simulink model "pinv_64x32"  (R2024a)
settings: Solver=VariableStepAuto  StartTime=0.0  StopTime=16384  RelTol=1e-3
PostLoadFcn:
  | xmcCheckSlxPath(bdroot)
  | setup
values from neighbouring files (symbols this model uses):
  MATMULT_RH_INPUT1_SAMPLES = MATMULT_INPUT_SAMPLES    (= 2048)    [setup.m]
undefined symbols (not defined in the file or in its folder): S, vsva2197, xcvc1902
libraries: aieBasic x7, dspsrcs4 x1, vmcUtilities x1, dspinverses x1, aieUtilities x1
settings Model: Creator=viswanad  LastModifiedBy=sdegala
settings SolverCC: AlgebraicLoopSolver=TrustRegion
settings DebuggingCC: UnconnectedInputMsg=warning  UnconnectedOutputMsg=warning  UnconnectedLineMsg=warning
settings ModelReferenceCC: EnableRefExpFcnMdlSchedulingChecks=on
settings RTWCC: GPUComputeCapability=3.5  DLArmComputeVersion=19.05

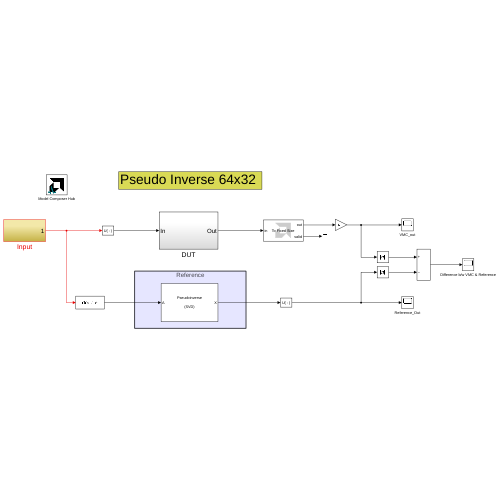
[thumbnail: Simulink's stored preview of the top-level diagram]
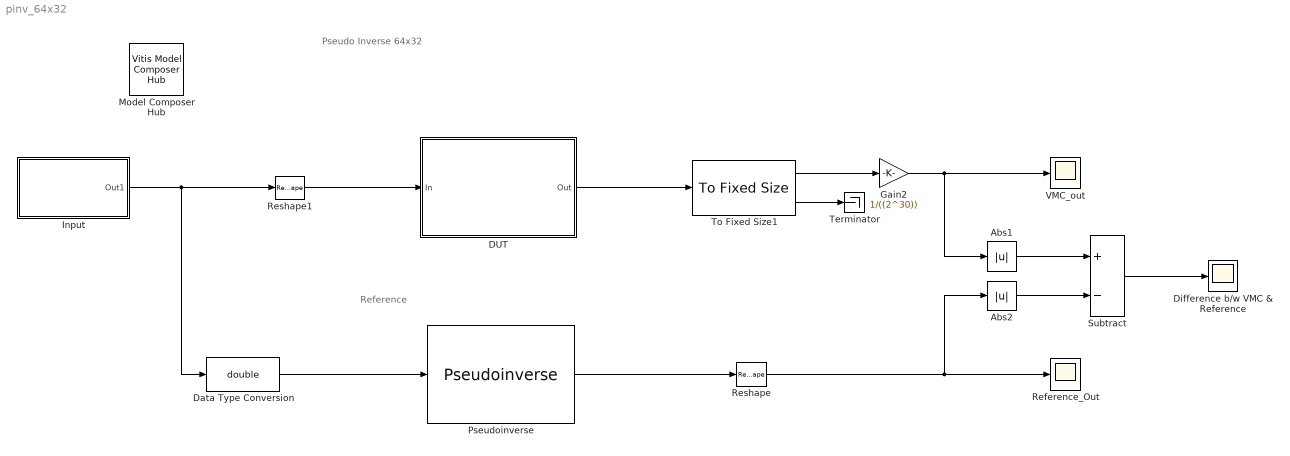
== system pinv_64x32 ==
  note: Reference
  note: Pseudo Inverse 64x32
  Abs1 : Abs  SaturateOnIntegerOverflow=off
  Abs2 : Abs  SaturateOnIntegerOverflow=off
  DUT : Subsystem
  Data Type Conversion : DataTypeConversion  OutDataTypeStr=double  SaturateOnIntegerOverflow=off  RndMeth=Floor
  Difference b/w VMC & Reference : Scope
  Gain2 : Gain  Gain=1/((2^30))  OutDataTypeStr=double
  Input : Subsystem
  Model Composer Hub : vmcUtilities/Vitis Model Composer Hub  Tag=genX  CodeGeneration=off  SubsystemName=DUT  BlockHierPath=pinv_64x32/DUT  SubsystemType=AIENode  AIEArrayConfig=Use entire AIE array  StartColumn=1  NumberOfColumns=1  TargetDirectory=./code  exportDesign=off  analyzeDesign=on  validateDesignOnHw=off  ExportType=AI Engines  IpVendor=xilinx.com  IpLibrary=hls  IpVersion=1.0  IpHWLanguage=Verilog  AieCompilerOptions={}  AieSimulatorOptions={}  CreateTestbench=on  TestbenchStackSize=10  RunRtlSim=off  RunCSim=off  RunAieSim=on  AieSimTimeout=50000  RunAieSimProfiling=off  LaunchVitisAnalyzer=off  PlotOutput=on  RunX86Sim=off  X86SimTimeout=10  GenHwImage=off  GenLibadfXo=off  GenHwValidationCode=off  PlatformType=Not Specified  HwSystemType=Baremetal  HwValidationTarget=hw  ProjDevice=xcvc1902-vsva2197-1LP-e-S  ProjDevicePart=xcvc1902-vsva2197-1LP-e-S  AIEType=AIE  SamplePeriod=-1  ClockFrequency=200  DataPathParallelism=1  xilinxfamily=versalaicore  part=xcvc1902  speed=-2MP-e-S  package=vsva2197  directory=./netlist  testbench=off  incr_netlist=off  synthesis_tool=Vivado  clock_wrapper=Clock Enables  dbl_ovrd=According to Block Masks  dcm_input_clock_period=10  sysclk_period=10  simulink_period=1  eval_field=0  IPInfoJsonString="{\"DUTSubsystemName\":\"DUT\",\"AIESubsystem\":{\"SubsystemName\":\"DUT\",\"TargetDirectory\":\"./code\",\"AIEArrayConfig\":\"Use entire AIE array\",\"StartColumn\":\"0\",\"NumberOfColumns\":\"1\"},\"SubsystemTag\":\"AIENode\"}"  LogFileName=/group/xcoswmktg2/robg/git/vmc_examples/github/Examples/AIENGINE/Pseudo_Inverse_64x32/code/model_composer.log  NThreads=4  IPConfigFile=/tmp/vmctmp-14485496486285087697/pinv_64x32_ipconfig.json
  Pseudoinverse : dspinverses/Pseudoinverse  wanterr=off  SimulateUsing=Interpreted execution
  Reference_Out : Scope
  Reshape : Reshape
  Reshape1 : Reshape
  Subtract : Sum  Inputs=+-
  Terminator : Terminator
  To Fixed Size1 : aieUtilities/To Fixed Size  Mode=Produce a valid output signal  OutputSize=2048  CopyMethod=Buffer samples to form output  HasStatusOutput=off
  VMC_out : Scope
  wires:
  Pseudoinverse/1 -> Reshape/1
  To Fixed Size1/1 -> Gain2/1
  Subtract/1 -> Difference b/w VMC & Reference/1
  Data Type Conversion/1 -> Pseudoinverse/1
  To Fixed Size1/2 -> Terminator/1
  Gain2/1 -> VMC_out/1, Abs1/1
  Reshape/1 -> Reference_Out/1, Abs2/1
  Abs1/1 -> Subtract/1
  Abs2/1 -> Subtract/2
  DUT/1(Out) -> To Fixed Size1/1
  Input/1(Out1) -> Reshape1/1, Data Type Conversion/1
  Reshape1/1 -> DUT/1(In)

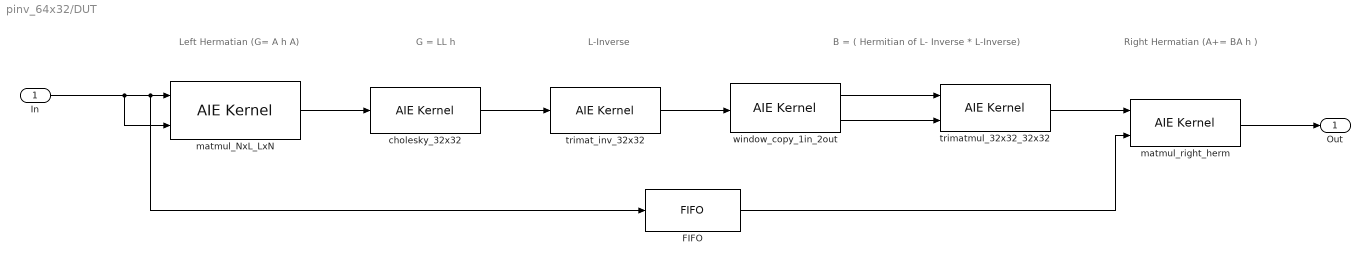
== system pinv_64x32/DUT ==
  note: Left Hermatian (G= A h A)
  note: G = LL h
  note: L-Inverse
  note: B = ( Hermitian of L- Inverse * L-Inverse)
  note: Right Hermatian (A+= BA h )
  In : Inport
  FIFO : aieBasic/FIFO  FifoDepth=MATMULT_RH_INPUT1_SAMPLES*3  FIFOType=0  TileType=0  RowLocation=0  ColLocation=0  channel=0  blockJsonConstraints=[]  deprecateConstraints=0
  cholesky_32x32 : aieBasic/AIE Kernel  KernelAllAttrs=s[12;12;9;9;19;14;21;23;24;21;12;24;26;26;26;27;28;9;21;23;23;23;24;25;14;19;19;29]@FunctionNameDeclFileNamePortNamesPortTypesPortSerializedTypesPortDirectionsPortWindowSizeEnablesPortWindowMarginEnablesPortSynchronicityEnablesPortSignalSizeEnablesFunctionDeclFunctionTemplateSpecKindFunctionTemplateParamNamesFunctionTemplateParamKindsFunctionTemplateParamTypesFunctionTemplateParamValuesFunctionTemplateParamEnablesClassDeclClassTemplateSpecKindClassTemplateParamNamesClassTemplateParamKindsClassTemplateParamTypesClassTemplateParamValuesClassTemplateParamEnablesClassCtorDeclsClassCtorParamNamesClassCtorParamTypesClassCtorParamSerializedTypes[1 1]@C[28 1]@t14@cholesky_32x32t49@../../../../../../baseband/inc/baseband_kernels.hC[2 1]@t5@inpktt6@outpktC[2 1]@t30@input_window_cint16 * restrictt31@output_window_cint16 * restrictC[2 1]@t37@{Q2{P{Tinput_window{1{t{Scint16}}}}}}t38@{Q2{P{Toutput_window{1{t{Scint16}}}}}}C[2 1]@t5@inputt6@outputC[2 1]@l1@l1@C[2 1]@l1@l0@C[2 1]@l1@l1@C[2 1]@l0@l0@t97@void cholesky_32x32(input_window_cint16 * restrict inpkt, output_window_cint16 * restrict outpkt)t4@nonee[0 1]@e[0 1]@e[0 1]@e[0 1]@e[0 1]@nne[0 1]@e[0 1]@e[0 1]@e[0 1]@e[0 1]@e[0 1]@e[0 1]@e[0 1]@e[0 1]@  PortNames={'inpkt'; 'outpkt'}  PortSerializedTypes={'{Q2{P{Tinput_window{1{t{Scint16}}}}}}'; '{Q2{P{Toutput_window{1{t{Scint16}}}}}}'}  PortWindowSizes={5.760000000000000000e+02, 5.760000000000000000e+02}  PortWindowMargins={0.000000000000000000e+00, 0.000000000000000000e+00}  PortSynchronicities={'sync', 'sync'}  PortSignalSizes={0.000000000000000000e+00; 0.000000000000000000e+00}  FunctionTemplateSpecKind=none  FunctionTemplateParamNames={}  FunctionTemplateParamKinds={}  FunctionTemplateParamTypes={}  FunctionTemplateParamValues={}  FunctionIndex=1  FunctionTabVisible=on  FunctionTemplateParamsVisible=off  FunctionDeclTypeOptions=C[1 1]@t97@void cholesky_32x32(input_window_cint16 * restrict inpkt, output_window_cint16 * restrict outpkt)  FunctionDecl=void cholesky_32x32(input_window_cint16 * restrict inpkt, output_window_cint16 * restrict outpkt)  FunctionTemplateParams={}  FunctionTemplateParamsEnables={}  PortAttrs={ 'input', 'inpkt', 'input_window_cint16 * restrict', 'CHOLESKY_32x32_INPUT_SAMPLES', '0', 'sync', ''; 'output', 'outpkt', 'output_window_cint16 * restrict', 'LINV_INPUT_SAMPLES', '', 'sync', '' }  PortAttrsEnables={'off', 'off', 'off', 'on', 'on', 'on', 'off';'off', 'off', 'off', 'on', 'off', 'on', 'off'}  SampleTime=-1  KernelHeaderFile=baseband_kernels.h  KernelFunction=cholesky_32x32  KernelInitFunction=chol_init  KernelSourceFile=cholesky_32x32.c  KernelSearchPaths={'kernels'}  PreProcOptions={}  blockJsonConstraints="{\"type\":\"constraint\",\"constraintType\":\"coreUtilization\",\"sid\":\"96\",\"lhs\":{\"type\":\"runtimeRatio\",\"args\":{\"type\":\"kernel\",\"name\":\"pinv_64x32/pinv64x32_sub/cholesky_32x32\",\"sid\":\"96\"}},\"rhs\":{\"type\":\"evaluable\",\"expr\":\"0.4\",\"value\":0.4},\"equality\":true}"
  matmul_NxL_LxN : aieBasic/AIE Kernel  KernelAllAttrs=s[12;12;9;9;19;14;21;23;21;23;24;21;15;17;12;24;26;26;26;27;28;9;21;23;23;23;24;25;14;19;19;29]@FunctionNameDeclFileNamePortNamesPortTypesPortSerializedTypesPortDirectionsPortWindowSizeEnablesPortWindowMarginEnablesPortBufferSizeEnablesPortBufferMarginEnablesPortSynchronicityEnablesPortSignalSizeEnablesPortBufferSizesPortBufferMarginsFunctionDeclFunctionTemplateSpecKindFunctionTemplateParamNamesFunctionTemplateParamKindsFunctionTemplateParamTypesFunctionTemplateParamValuesFunctionTemplateParamEnablesClassDeclClassTemplateSpecKindClassTemplateParamNamesClassTemplateParamKindsClassTemplateParamTypesClassTemplateParamValuesClassTemplateParamEnablesClassCtorDeclsClassCtorParamNamesClassCtorParamTypesClassCtorParamSerializedTypes[1 1]@C[32 1]@t14@matmul_NxL_LxNt28@../../kernels/blas_kernels.hC[3 1]@t4@matAt4@matBt4@matCC[3 1]@t30@input_window_cint16 * restrictt30@input_window_cint16 * restrictt31@output_window_cint16 * restrictC[3 1]@t37@{Q2{P{Tinput_window{1{t{Scint16}}}}}}t37@{Q2{P{Tinput_window{1{t{Scint16}}}}}}t38@{Q2{P{Toutput_window{1{t{Scint16}}}}}}C[3 1]@t5@inputt5@inputt6@outputC[3 1]@l1@l1@l1@C[3 1]@l1@l1@l0@C[3 1]@l0@l0@l0@C[3 1]@l0@l0@l0@C[3 1]@l1@l1@l1@C[3 1]@l0@l0@l0@C[3 1]@nnnC[3 1]@nnnt131@void matmul_NxL_LxN(input_window_cint16 * restrict matA, input_window_cint16 * restrict matB, output_window_cint16 * restrict matC)t4@nonee[0 1]@e[0 1]@e[0 1]@e[0 1]@e[0 1]@nne[0 1]@e[0 1]@e[0 1]@e[0 1]@e[0 1]@e[0 1]@e[0 1]@e[0 1]@e[0 1]@  PortNames={'matA'; 'matB'; 'matC'}  PortSerializedTypes={'{Q2{P{Tinput_window{1{t{Scint16}}}}}}'; '{Q2{P{Tinput_window{1{t{Scint16}}}}}}'; '{Q2{P{Toutput_window{1{t{Scint16}}}}}}'}  PortWindowSizes={2.048000000000000000e+03, 2.048000000000000000e+03, 5.760000000000000000e+02}  PortWindowMargins={0.000000000000000000e+00, 0.000000000000000000e+00, 0.000000000000000000e+00}  PortSynchronicities={'sync', 'sync', 'sync'}  PortSignalSizes={0.000000000000000000e+00; 0.000000000000000000e+00; 0.000000000000000000e+00}  FunctionTemplateSpecKind=none  FunctionTemplateParamNames={}  FunctionTemplateParamKinds={}  FunctionTemplateParamTypes={}  FunctionTemplateParamValues={}  FunctionIndex=1  FunctionTabVisible=on  FunctionTemplateParamsVisible=off  FunctionDeclTypeOptions=C[1 1]@t131@void matmul_NxL_LxN(input_window_cint16 * restrict matA, input_window_cint16 * restrict matB, output_window_cint16 * restrict matC)  FunctionDecl=void matmul_NxL_LxN(input_window_cint16 * restrict matA, input_window_cint16 * restrict matB, output_window_cint16 * restrict matC)  FunctionTemplateParams={}  FunctionTemplateParamsEnables={}  PortAttrs={ 'input', 'matA', 'input_window_cint16 * restrict', 'MATMULT_INPUT_SAMPLES', '0', 'sync', ''; 'input', 'matB', 'input_window_cint16 * restrict', 'MATMULT_INPUT_SAMPLES', '0', 'sync', ''; 'output', 'matC', 'output_window_cint16 * restrict', 'MATMULT_OUTPUT_SAMPLES', '', 'sync', '' }  PortAttrsEnables={'off', 'off', 'off', 'on', 'on', 'on', 'off';'off', 'off', 'off', 'on', 'on', 'on', 'off';'off', 'off', 'off', 'on', 'off', 'on', 'off'}  SampleTime=-1  KernelHeaderFile=blas_kernels.h  KernelFunction=matmul_NxL_LxN  KernelInitFunction=matmul_NxL_LxN_init  KernelSourceFile=matmul_NxL_LxN.cc  KernelSearchPaths={'kernels'}  PreProcOptions={}  blockJsonConstraints="[{\"type\":\"constraint\",\"constraintType\":\"coreUtilization\",\"sid\":\"95\",\"lhs\":{\"type\":\"runtimeRatio\",\"args\":{\"type\":\"kernel\",\"name\":\"pinv_64x32/pinv64x32_sub/matmul_NxL_LxN\",\"sid\":\"95\"}},\"rhs\":{\"type\":\"evaluable\",\"expr\":\"0.4\",\"value\":0.4},\"equality\":true},{\"type\":\"constraint\",\"constraintType\":\"location_kernel\",\"sid\":\"95\",\"lhs\":{\"type\":\"location\",\"templParam\":\"kernel\",\"args\":{\"type\":\"kernel\",\"name\":\"pinv_64x32/pinv64x32_sub/matmul_NxL_LxN\",\"sid\":\"95\"}},\"rhs\":{\"type\":\"location\",\"templParam\":\"kernel\",\"args\":{\"type\":\"kernel\",\"name\":\"pinv_64x32/pinv64x32_sub/cholesky_32x32\",\"sid\":\"96\"}},\"equality\":true}]"
  matmul_right_herm : aieBasic/AIE Kernel  KernelAllAttrs=s[12;12;9;9;19;14;21;23;21;23;24;21;15;17;12;24;26;26;26;27;28;9;21;23;23;23;24;25;14;19;19;29]@FunctionNameDeclFileNamePortNamesPortTypesPortSerializedTypesPortDirectionsPortWindowSizeEnablesPortWindowMarginEnablesPortBufferSizeEnablesPortBufferMarginEnablesPortSynchronicityEnablesPortSignalSizeEnablesPortBufferSizesPortBufferMarginsFunctionDeclFunctionTemplateSpecKindFunctionTemplateParamNamesFunctionTemplateParamKindsFunctionTemplateParamTypesFunctionTemplateParamValuesFunctionTemplateParamEnablesClassDeclClassTemplateSpecKindClassTemplateParamNamesClassTemplateParamKindsClassTemplateParamTypesClassTemplateParamValuesClassTemplateParamEnablesClassCtorDeclsClassCtorParamNamesClassCtorParamTypesClassCtorParamSerializedTypes[1 1]@C[32 1]@t17@matmul_right_hermt24@../../inc/blas_kernels.hC[3 1]@t4@matAt4@matBt4@matCC[3 1]@t30@input_window_cint16 * restrictt30@input_window_cint16 * restrictt31@output_window_cint16 * restrictC[3 1]@t37@{Q2{P{Tinput_window{1{t{Scint16}}}}}}t37@{Q2{P{Tinput_window{1{t{Scint16}}}}}}t38@{Q2{P{Toutput_window{1{t{Scint16}}}}}}C[3 1]@t5@inputt5@inputt6@outputC[3 1]@l1@l1@l1@C[3 1]@l1@l1@l0@C[3 1]@l0@l0@l0@C[3 1]@l0@l0@l0@C[3 1]@l1@l1@l1@C[3 1]@l0@l0@l0@C[3 1]@nnnC[3 1]@nnnt134@void matmul_right_herm(input_window_cint16 * restrict matA, input_window_cint16 * restrict matB, output_window_cint16 * restrict matC)t4@nonee[0 1]@e[0 1]@e[0 1]@e[0 1]@e[0 1]@nne[0 1]@e[0 1]@e[0 1]@e[0 1]@e[0 1]@e[0 1]@e[0 1]@e[0 1]@e[0 1]@  PortNames={'matA'; 'matB'; 'matC'}  PortSerializedTypes={'{Q2{P{Tinput_window{1{t{Scint16}}}}}}'; '{Q2{P{Tinput_window{1{t{Scint16}}}}}}'; '{Q2{P{Toutput_window{1{t{Scint16}}}}}}'}  PortWindowSizes={1.024000000000000000e+03, 2.048000000000000000e+03, 2.048000000000000000e+03}  PortWindowMargins={0.000000000000000000e+00, 0.000000000000000000e+00, 0.000000000000000000e+00}  PortSynchronicities={'sync', 'sync', 'sync'}  PortSignalSizes={0.000000000000000000e+00; 0.000000000000000000e+00; 0.000000000000000000e+00}  FunctionTemplateSpecKind=none  FunctionTemplateParamNames={}  FunctionTemplateParamKinds={}  FunctionTemplateParamTypes={}  FunctionTemplateParamValues={}  FunctionIndex=1  FunctionTabVisible=on  FunctionTemplateParamsVisible=off  FunctionDeclTypeOptions=C[1 1]@t134@void matmul_right_herm(input_window_cint16 * restrict matA, input_window_cint16 * restrict matB, output_window_cint16 * restrict matC)  FunctionDecl=void matmul_right_herm(input_window_cint16 * restrict matA, input_window_cint16 * restrict matB, output_window_cint16 * restrict matC)  FunctionTemplateParams={}  FunctionTemplateParamsEnables={}  PortAttrs={ 'input', 'matA', 'input_window_cint16 * restrict', 'TRIMULT_OUTPUT_SAMPLES', '', 'sync', ''; 'input', 'matB', 'input_window_cint16 * restrict', 'MATMULT_INPUT_SAMPLES', '', 'sync', ''; 'output', 'matC', 'output_window_cint16 * restrict', 'MATMULT_INPUT_SAMPLES', '', 'sync', '' }  PortAttrsEnables={'off', 'off', 'off', 'on', 'on', 'on', 'off';'off', 'off', 'off', 'on', 'on', 'on', 'off';'off', 'off', 'off', 'on', 'off', 'on', 'off'}  SampleTime=-1  KernelHeaderFile=blas_kernels.h  KernelFunction=matmul_right_herm  KernelSourceFile=matmul_right_herm.cc  KernelSearchPaths={'kernels'}  PreProcOptions={}  blockJsonConstraints="{\"type\":\"constraint\",\"constraintType\":\"coreUtilization\",\"sid\":\"100\",\"lhs\":{\"type\":\"runtimeRatio\",\"args\":{\"type\":\"kernel\",\"name\":\"pinv_64x32/pinv64x32_sub/matmul_right_herm\",\"sid\":\"100\"}},\"rhs\":{\"type\":\"evaluable\",\"expr\":\"0.75\",\"value\":0.75},\"equality\":true}"
  trimat_inv_32x32 : aieBasic/AIE Kernel  KernelAllAttrs=s[12;12;9;9;19;14;21;23;24;21;12;24;26;26;26;27;28;9;21;23;23;23;24;25;14;19;19;29]@FunctionNameDeclFileNamePortNamesPortTypesPortSerializedTypesPortDirectionsPortWindowSizeEnablesPortWindowMarginEnablesPortSynchronicityEnablesPortSignalSizeEnablesFunctionDeclFunctionTemplateSpecKindFunctionTemplateParamNamesFunctionTemplateParamKindsFunctionTemplateParamTypesFunctionTemplateParamValuesFunctionTemplateParamEnablesClassDeclClassTemplateSpecKindClassTemplateParamNamesClassTemplateParamKindsClassTemplateParamTypesClassTemplateParamValuesClassTemplateParamEnablesClassCtorDeclsClassCtorParamNamesClassCtorParamTypesClassCtorParamSerializedTypes[1 1]@C[28 1]@t16@trimat_inv_32x32t41@../../../../../../blas/inc/blas_kernels.hC[2 1]@t4@L_int5@x_outC[2 1]@t21@input_window_cint16 *t22@output_window_cint16 *C[2 1]@t33@{P{Tinput_window{1{t{Scint16}}}}}t34@{P{Toutput_window{1{t{Scint16}}}}}C[2 1]@t5@inputt6@outputC[2 1]@l1@l1@C[2 1]@l1@l0@C[2 1]@l1@l1@C[2 1]@l0@l0@t79@void trimat_inv_32x32(input_window_cint16 * L_in, output_window_cint16 * x_out)t4@nonee[0 1]@e[0 1]@e[0 1]@e[0 1]@e[0 1]@nne[0 1]@e[0 1]@e[0 1]@e[0 1]@e[0 1]@e[0 1]@e[0 1]@e[0 1]@e[0 1]@  PortNames={'L_in'; 'x_out'}  PortSerializedTypes={'{P{Tinput_window{1{t{Scint16}}}}}'; '{P{Toutput_window{1{t{Scint16}}}}}'}  PortWindowSizes={5.760000000000000000e+02, 6.400000000000000000e+02}  PortWindowMargins={0.000000000000000000e+00, 0.000000000000000000e+00}  PortSynchronicities={'sync', 'sync'}  PortSignalSizes={0.000000000000000000e+00; 0.000000000000000000e+00}  FunctionTemplateSpecKind=none  FunctionTemplateParamNames={}  FunctionTemplateParamKinds={}  FunctionTemplateParamTypes={}  FunctionTemplateParamValues={}  FunctionIndex=1  FunctionTabVisible=on  FunctionTemplateParamsVisible=off  FunctionDeclTypeOptions=C[1 1]@t79@void trimat_inv_32x32(input_window_cint16 * L_in, output_window_cint16 * x_out)  FunctionDecl=void trimat_inv_32x32(input_window_cint16 * L_in, output_window_cint16 * x_out)  FunctionTemplateParams={}  FunctionTemplateParamsEnables={}  PortAttrs={ 'input', 'L_in', 'input_window_cint16 *', 'LINV_INPUT_SAMPLES', '0', 'sync', ''; 'output', 'x_out', 'output_window_cint16 *', 'LINV_OUTPUT_SAMPLES', '', 'sync', '' }  PortAttrsEnables={'off', 'off', 'off', 'on', 'on', 'on', 'off';'off', 'off', 'off', 'on', 'off', 'on', 'off'}  SampleTime=-1  KernelHeaderFile=blas_kernels.h  KernelFunction=trimat_inv_32x32  KernelInitFunction=trimat_inv_32x32_init  KernelSourceFile=trimat_inv_32x32.cc  KernelSearchPaths={'kernels'}  PreProcOptions={}  blockJsonConstraints="{\"type\":\"constraint\",\"constraintType\":\"coreUtilization\",\"sid\":\"97\",\"lhs\":{\"type\":\"runtimeRatio\",\"args\":{\"type\":\"kernel\",\"name\":\"pinv_64x32/pinv64x32_sub/trimat_inv_32x32\",\"sid\":\"97\"}},\"rhs\":{\"type\":\"evaluable\",\"expr\":\"0.8\",\"value\":0.8},\"equality\":true}"
  trimatmul_32x32_32x32 : aieBasic/AIE Kernel  KernelAllAttrs=s[12;12;9;9;19;14;21;23;24;21;12;24;26;26;26;27;28;9;21;23;23;23;24;25;14;19;19;29]@FunctionNameDeclFileNamePortNamesPortTypesPortSerializedTypesPortDirectionsPortWindowSizeEnablesPortWindowMarginEnablesPortSynchronicityEnablesPortSignalSizeEnablesFunctionDeclFunctionTemplateSpecKindFunctionTemplateParamNamesFunctionTemplateParamKindsFunctionTemplateParamTypesFunctionTemplateParamValuesFunctionTemplateParamEnablesClassDeclClassTemplateSpecKindClassTemplateParamNamesClassTemplateParamKindsClassTemplateParamTypesClassTemplateParamValuesClassTemplateParamEnablesClassCtorDeclsClassCtorParamNamesClassCtorParamTypesClassCtorParamSerializedTypes[1 1]@C[28 1]@t21@trimatmul_32x32_32x32t41@../../../../../../blas/inc/blas_kernels.hC[3 1]@t4@matAt4@matBt4@matCC[3 1]@t30@input_window_cint16 * restrictt30@input_window_cint16 * restrictt31@output_window_cint16 * restrictC[3 1]@t37@{Q2{P{Tinput_window{1{t{Scint16}}}}}}t37@{Q2{P{Tinput_window{1{t{Scint16}}}}}}t38@{Q2{P{Toutput_window{1{t{Scint16}}}}}}C[3 1]@t5@inputt5@inputt6@outputC[3 1]@l1@l1@l1@C[3 1]@l1@l1@l0@C[3 1]@l1@l1@l1@C[3 1]@l0@l0@l0@t138@void trimatmul_32x32_32x32(input_window_cint16 * restrict matA, input_window_cint16 * restrict matB, output_window_cint16 * restrict matC)t4@nonee[0 1]@e[0 1]@e[0 1]@e[0 1]@e[0 1]@nne[0 1]@e[0 1]@e[0 1]@e[0 1]@e[0 1]@e[0 1]@e[0 1]@e[0 1]@e[0 1]@  PortNames={'matA'; 'matB'; 'matC'}  PortSerializedTypes={'{Q2{P{Tinput_window{1{t{Scint16}}}}}}'; '{Q2{P{Tinput_window{1{t{Scint16}}}}}}'; '{Q2{P{Toutput_window{1{t{Scint16}}}}}}'}  PortWindowSizes={6.400000000000000000e+02, 6.400000000000000000e+02, 1.024000000000000000e+03}  PortWindowMargins={0.000000000000000000e+00, 0.000000000000000000e+00, 0.000000000000000000e+00}  PortSynchronicities={'sync', 'sync', 'sync'}  PortSignalSizes={0.000000000000000000e+00; 0.000000000000000000e+00; 0.000000000000000000e+00}  FunctionTemplateSpecKind=none  FunctionTemplateParamNames={}  FunctionTemplateParamKinds={}  FunctionTemplateParamTypes={}  FunctionTemplateParamValues={}  FunctionIndex=1  FunctionTabVisible=on  FunctionTemplateParamsVisible=off  FunctionDeclTypeOptions=C[1 1]@t138@void trimatmul_32x32_32x32(input_window_cint16 * restrict matA, input_window_cint16 * restrict matB, output_window_cint16 * restrict matC)  FunctionDecl=void trimatmul_32x32_32x32(input_window_cint16 * restrict matA, input_window_cint16 * restrict matB, output_window_cint16 * restrict matC)  FunctionTemplateParams={}  FunctionTemplateParamsEnables={}  PortAttrs={ 'input', 'matA', 'input_window_cint16 * restrict', 'TRIMULT_INPUT_SAMPLES', '0', 'sync', ''; 'input', 'matB', 'input_window_cint16 * restrict', 'TRIMULT_INPUT_SAMPLES', '0', 'sync', ''; 'output', 'matC', 'output_window_cint16 * restrict', 'MATMULT_RH_INPUT0_SAMPLES', '', 'sync', '' }  PortAttrsEnables={'off', 'off', 'off', 'on', 'on', 'on', 'off';'off', 'off', 'off', 'on', 'on', 'on', 'off';'off', 'off', 'off', 'on', 'off', 'on', 'off'}  SampleTime=-1  KernelHeaderFile=blas_kernels.h  KernelFunction=trimatmul_32x32_32x32  KernelSourceFile=trimatmul_32x32_32x32.cc  KernelSearchPaths={'kernels'}  PreProcOptions={}  blockJsonConstraints="{\"type\":\"constraint\",\"constraintType\":\"coreUtilization\",\"sid\":\"98\",\"lhs\":{\"type\":\"runtimeRatio\",\"args\":{\"type\":\"kernel\",\"name\":\"pinv_64x32/pinv64x32_sub/trimatmul_32x32_32x32\",\"sid\":\"98\"}},\"rhs\":{\"type\":\"evaluable\",\"expr\":\"0.8\",\"value\":0.8},\"equality\":true}"
  window_copy_1in_2out : aieBasic/AIE Kernel  KernelAllAttrs=s[12;12;9;9;19;14;21;23;21;23;24;21;15;17;12;24;26;26;26;27;28;9;21;23;23;23;24;25;14;19;19;29]@FunctionNameDeclFileNamePortNamesPortTypesPortSerializedTypesPortDirectionsPortWindowSizeEnablesPortWindowMarginEnablesPortBufferSizeEnablesPortBufferMarginEnablesPortSynchronicityEnablesPortSignalSizeEnablesPortBufferSizesPortBufferMarginsFunctionDeclFunctionTemplateSpecKindFunctionTemplateParamNamesFunctionTemplateParamKindsFunctionTemplateParamTypesFunctionTemplateParamValuesFunctionTemplateParamEnablesClassDeclClassTemplateSpecKindClassTemplateParamNamesClassTemplateParamKindsClassTemplateParamTypesClassTemplateParamValuesClassTemplateParamEnablesClassCtorDeclsClassCtorParamNamesClassCtorParamTypesClassCtorParamSerializedTypes[1 1]@C[32 1]@t20@window_copy_1in_2outt18@../../inc/common.hC[3 1]@t8@cb_inputt10@cb_output0t10@cb_output1C[3 1]@t47@adf::input_circular_buffer< cint16 > & restrictt48@adf::output_circular_buffer< cint16 > & restrictt48@adf::output_circular_buffer< cint16 > & restrictC[3 1]@t51@{Q2{R{Tadf::input_circular_buffer{1{t{Scint16}}}}}}t52@{Q2{R{Tadf::output_circular_buffer{1{t{Scint16}}}}}}t52@{Q2{R{Tadf::output_circular_buffer{1{t{Scint16}}}}}}C[3 1]@t5@inputt6@outputt6@outputC[3 1]@l1@l1@l1@C[3 1]@l1@l0@l0@C[3 1]@l1@l1@l1@C[3 1]@l0@l0@l0@C[3 1]@l1@l1@l1@C[3 1]@l0@l0@l0@C[3 1]@nnnC[3 1]@nnnt205@void window_copy_1in_2out(adf::input_circular_buffer< cint16 > & restrict cb_input, adf::output_circular_buffer< cint16 > & restrict cb_output0, adf::output_circular_buffer< cint16 > & restrict cb_output1)t4@nonee[0 1]@e[0 1]@e[0 1]@e[0 1]@e[0 1]@nne[0 1]@e[0 1]@e[0 1]@e[0 1]@e[0 1]@e[0 1]@e[0 1]@e[0 1]@e[0 1]@  PortNames={'cb_input'; 'cb_output0'; 'cb_output1'}  PortSerializedTypes={'{Q2{R{Tadf::input_circular_buffer{1{t{Scint16}}}}}}'; '{Q2{R{Tadf::output_circular_buffer{1{t{Scint16}}}}}}'; '{Q2{R{Tadf::output_circular_buffer{1{t{Scint16}}}}}}'}  PortWindowSizes={6.400000000000000000e+02, 6.400000000000000000e+02, 6.400000000000000000e+02}  PortWindowMargins={0.000000000000000000e+00, 0.000000000000000000e+00, 0.000000000000000000e+00}  PortSynchronicities={'sync', 'sync', 'sync'}  PortSignalSizes={0.000000000000000000e+00; 0.000000000000000000e+00; 0.000000000000000000e+00}  FunctionTemplateSpecKind=none  FunctionTemplateParamNames={}  FunctionTemplateParamKinds={}  FunctionTemplateParamTypes={}  FunctionTemplateParamValues={}  FunctionIndex=1  FunctionTabVisible=on  FunctionTemplateParamsVisible=off  FunctionDeclTypeOptions=C[1 1]@t208@void window_copy_1in_2out(adf::input_circular_buffer< cint16 > && restrict cb_input, adf::output_circular_buffer< cint16 > && restrict cb_output0, adf::output_circular_buffer< cint16 > && restrict cb_output1)  FunctionDecl=void window_copy_1in_2out(adf::input_circular_buffer< cint16 > && restrict cb_input, adf::output_circular_buffer< cint16 > && restrict cb_output0, adf::output_circular_buffer< cint16 > && restrict cb_output1)  FunctionTemplateParams={}  FunctionTemplateParamsEnables={}  PortAttrs={ 'input', 'cb_input', 'adf::input_circular_buffer< cint16 > & restrict', 'TRIMULT_INPUT_SAMPLES ', '0', 'sync', ''; 'output', 'cb_output0', 'adf::output_circular_buffer< cint16 > & restrict', 'TRIMULT_INPUT_SAMPLES ', '', 'sync', ''; 'output', 'cb_output1', 'adf::output_circular_buffer< cint16 > & restrict', 'TRIMULT_INPUT_SAMPLES ', '', 'sync', '' }  PortAttrsEnables={'off', 'off', 'off', 'on', 'off', 'off', 'off';'off', 'off', 'off', 'on', 'off', 'off', 'off';'off', 'off', 'off', 'on', 'off', 'off', 'off'}  SampleTime=-1  KernelHeaderFile=common.h  KernelFunction=window_copy_1in_2out  KernelSourceFile=window_copy_1in_2out.cc  KernelSearchPaths={'kernels'}  PreProcOptions={}  blockJsonConstraints="[{\"type\":\"constraint\",\"constraintType\":\"coreUtilization\",\"sid\":\"99\",\"lhs\":{\"type\":\"runtimeRatio\",\"args\":{\"type\":\"kernel\",\"name\":\"pinv_64x32/pinv64x32_sub/window_copy_1in_2out1\",\"sid\":\"99\"}},\"rhs\":{\"type\":\"evaluable\",\"expr\":\"0.1\",\"value\":0.1},\"equality\":true},{\"type\":\"constraint\",\"constraintType\":\"location_kernel\",\"sid\":\"99\",\"lhs\":{\"type\":\"location\",\"templParam\":\"kernel\",\"args\":{\"type\":\"kernel\",\"name\":\"pinv_64x32/pinv64x32_sub/window_copy_1in_2out1\",\"sid\":\"99\"}},\"rhs\":{\"type\":\"location\",\"templParam\":\"kernel\",\"args\":{\"type\":\"kernel\",\"name\":\"pinv_64x32/pinv64x32_sub/trimatmul_32x32_32x32\",\"sid\":\"98\"}},\"equality\":true}]"
  Out : Outport
  wires:
  matmul_NxL_LxN/1 -> cholesky_32x32/1
  cholesky_32x32/1 -> trimat_inv_32x32/1
  trimat_inv_32x32/1 -> window_copy_1in_2out/1
  window_copy_1in_2out/1 -> trimatmul_32x32_32x32/1
  window_copy_1in_2out/2 -> trimatmul_32x32_32x32/2
  trimatmul_32x32_32x32/1 -> matmul_right_herm/1
  In/1 -> FIFO/1, matmul_NxL_LxN/1, matmul_NxL_LxN/2
  matmul_right_herm/1 -> Out/1
  FIFO/1 -> matmul_right_herm/2

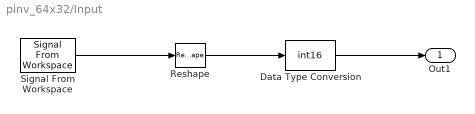
== system pinv_64x32/Input ==
  Data Type Conversion : DataTypeConversion  OutDataTypeStr=int16  SaturateOnIntegerOverflow=off  RndMeth=Floor
  Reshape : Reshape  OutputDimensionality=Customize  OutputDimensions=[64,32]
  Signal From Workspace : dspsrcs4/Signal From Workspace  X=input_data  Ts=1  nsamps=2048  OutputAfterFinalValue=Setting to zero  ignoreOrWarnInputAndFrameLengths=off  OutputFrames=off
  Out1 : Outport  VectorParamsAs1DForOutWhenUnconnected=off
  wires:
  Signal From Workspace/1 -> Reshape/1
  Data Type Conversion/1 -> Out1/1
  Reshape/1 -> Data Type Conversion/1
